simulink model "refGenerator"  (R2019b)
settings: Solver=ode8  StartTime=0.0  StopTime=120  FixedStep=0.01  RelTol=1e-3
libraries: simulink x1
settings Model: Creator=maxva  LastModifiedBy=maxva

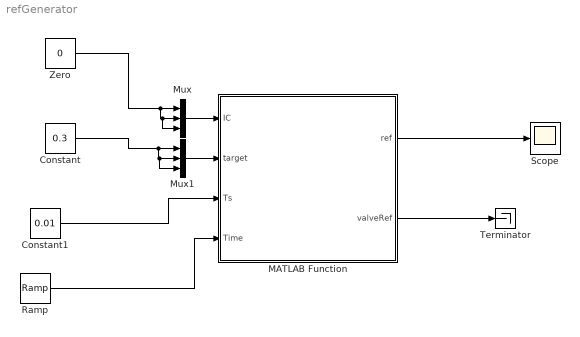
== system refGenerator ==
  Constant : Constant  Value=0.3
  Constant1 : Constant  Value=0.01
  MATLAB Function : MATLAB Function  TreatAsAtomicUnit=on
  Mux : Mux  Inputs=3
  Mux1 : Mux  Inputs=3
  Ramp : simulink/Sources/Ramp  slope=1  start=0  InitialOutput=0
  Scope : Scope
  Terminator : Terminator
  Zero : Constant  Value=0  OutDataTypeStr=Inherit: Inherit via back propagation
  wires:
  MATLAB Function/1(ref) -> Scope/1
  MATLAB Function/2(valveRef) -> Terminator/1
  Constant1/1 -> MATLAB Function/3(Ts)
  Ramp/1 -> MATLAB Function/4(Time)
  Mux1/1 -> MATLAB Function/2(target)
  Mux/1 -> MATLAB Function/1(IC)
  Zero/1 -> Mux/3, Mux/2, Mux/1
  Constant/1 -> Mux1/3, Mux1/2, Mux1/1

== matlab function refGenerator/MATLAB Function ==
  data: IC input; ref output; target input; valveRef output; Ts input; Time input
function [ref, valveRef] = fcn(IC, target,Ts,Time)
% input: IC, 3D vector of initial conditions of system
% input: target, 3D vector of target reference for fluid  heights
% input: Sampling time Ts

% output: ref, 3*1 vector containing fluid height references 
% output: valveRef, 2*1 vector containg valve references. Needed for MPC,
% can be ignored (use terminator block in simulink)

%% constants
Atank = 0.0154;
uMaxL = 0.1;        % from Bart's work
uMaxR =  0.09;      % from Bart's work
%% reshaping (check gode generation?)
IC = reshape(IC, [],1);             %  force IC to be a vector
target = reshape(target, [],1);     %  idem
%% calculations
tf = 1.1*sum(target)*Atank/(uMaxL+uMaxR-3*0.01)*1000;  % give a 10% margin for pump dynamics etc, choose 50% of maximum disturbance allowed as 'constant disturbance'
ref = zeros(3,1);
valveRef = zeros(2,1);
matr = [1 zeros(1,3);
        0 1  0    0;
        1 tf tf^2 tf^3;
        0 1 2*tf 3*tf^2];
invmatr = inv(matr);
if  Time < tf
    for i =1:3
        vec = [IC(i);0;target(i);0];
        polyCoeff = invmatr*vec;
        ref(i,1) = polyCoeff(1)+polyCoeff(2)*Time+polyCoeff(3)*Time.^2+polyCoeff(4)*Time.^3;
    end
else
    ref = target;
end
